simulink model "gimbal_quats_n_stuff"  (R2016a)
settings: Solver=FixedStepAuto  StartTime=0.0  StopTime=10.0  FixedStep=1e-3  RelTol=1e-3
libraries: aerolibtransform2 x4
settings Model: Creator=glenn  LastModifiedBy=glenn
settings GRTTargetCC: GeneratePreprocessorConditionals=Use local settings

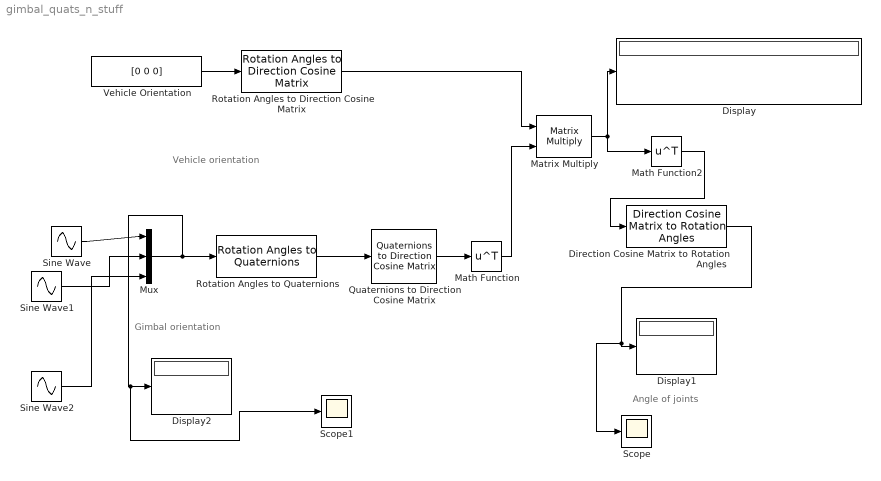
== system gimbal_quats_n_stuff ==
  note: Vehicle orientation
  note: Gimbal orientation
  note: Angle of joints
  Direction Cosine Matrix to Rotation Angles : aerolibtransform2/Direction Cosine Matrix to Rotation Angles  rotationOrder=ZXZ  lim=ZeroR3
      settings: AttributesFormatString=Rotation Order: %<rotationOrder>
  Display : Display
  Display1 : Display
  Display2 : Display
  Math Function : Math  Operator=transpose  SaturateOnIntegerOverflow=on
  Math Function2 : Math  Operator=transpose  SaturateOnIntegerOverflow=on
  Matrix Multiply : Product  Multiplication=Matrix(*)
  Mux : Mux  Inputs=3
  Quaternions to Direction Cosine Matrix : aerolibtransform2/Quaternions to  Direction Cosine Matrix
  Rotation Angles to Direction Cosine Matrix : aerolibtransform2/Rotation Angles to Direction Cosine Matrix  rotationOrder=ZYX
  Rotation Angles to Quaternions : aerolibtransform2/Rotation Angles to Quaternions  rotationOrder=ZXZ
  Scope : Scope
  Scope1 : Scope
  Sine Wave : Sin  Amplitude=pi  SampleTime=0
  Sine Wave1 : Sin  Amplitude=pi/2  Bias=pi/2  SampleTime=0
  Sine Wave2 : Sin  Amplitude=pi/2  Bias=-pi/2  SampleTime=0
  Vehicle Orientation : Constant  Value=[0 0 0]
  wires:
  Mux/1 -> Scope1/1, Display2/1, Rotation Angles to Quaternions/1
  Rotation Angles to Quaternions/1 -> Quaternions to Direction Cosine Matrix/1
  Vehicle Orientation/1 -> Rotation Angles to Direction Cosine Matrix/1
  Matrix Multiply/1 -> Math Function2/1, Display/1
  Direction Cosine Matrix to Rotation Angles/1 -> Scope/1, Display1/1
  Quaternions to Direction Cosine Matrix/1 -> Math Function/1
  Math Function/1 -> Matrix Multiply/2
  Rotation Angles to Direction Cosine Matrix/1 -> Matrix Multiply/1
  Math Function2/1 -> Direction Cosine Matrix to Rotation Angles/1
  Sine Wave/1 -> Mux/1
  Sine Wave1/1 -> Mux/2
  Sine Wave2/1 -> Mux/3
